simulink model "step_input_Q3_standard"  (R2023a)
settings: Solver=VariableStepAuto  StartTime=0.0  StopTime=50  RelTol=1e-3
libraries: simulink_extras x2
settings Model: Creator=anshu  LastModifiedBy=anshu

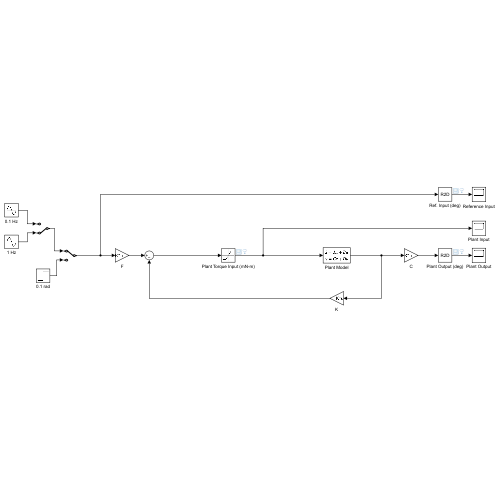
[thumbnail: Simulink's stored preview of the top-level diagram]
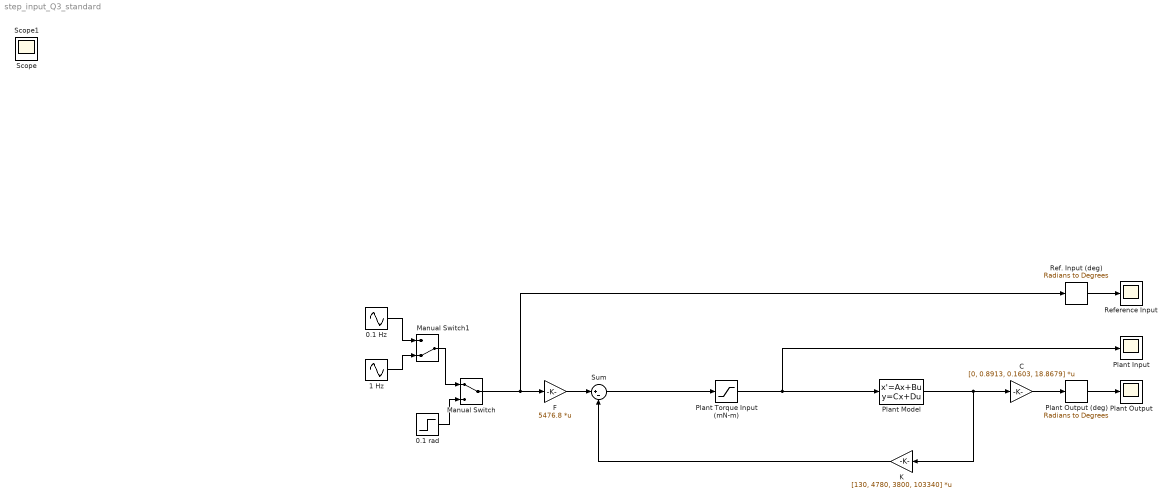
== system step_input_Q3_standard ==
  0.1 Hz : Sin  Amplitude=2.5  Frequency=0.628  SampleTime=0
  0.1 rad : Step  After=0.1  SampleTime=0
  1 Hz : Sin  Amplitude=0.3  Frequency=6.28  SampleTime=0
  C : Gain  Gain=[0, 0.8913, 0.1603, 18.8679]  Multiplication=Matrix(K*u)
  F : Gain  Gain=5476.8  Multiplication=Matrix(K*u)
  K : Gain  Gain=[130, 4780, 3800, 103340]  Multiplication=Matrix(K*u)
  Manual Switch : ManualSwitch
  Manual Switch1 : ManualSwitch  CurrentSetting=0
  Plant Input : Scope
  Plant Model : StateSpace  A=[-5.2954, -70.1022, -343.1258, 0; 1, 0, 0, 0; 0, 1, 0, 0; 0, 0, 1, 0]  B=[1; 0; 0; 0]  C=eye(4)  D=zeros(4,1)  InitialCondition=0  ParameterTunability=Unconstrained
  Plant Output : Scope
  Plant Output (deg) : simulink_extras/Transformations/Radians to Degrees
  Plant Torque Input (mN-m) : Saturate  UpperLimit=67  LowerLimit=-67
  Ref. Input (deg) : simulink_extras/Transformations/Radians to Degrees
  Reference Input : Scope
  Sum : Sum  Inputs=|+-
  Scope : Scope
  Scope1 : Scope
  wires:
  F/1 -> Sum/1
  Sum/1 -> Plant Torque Input (mN-m)/1
  Plant Model/1 -> C/1, K/1
  K/1 -> Sum/2
  Plant Torque Input (mN-m)/1 -> Plant Input/1, Plant Model/1
  C/1 -> Plant Output (deg)/1
  Plant Output (deg)/1 -> Plant Output/1
  Ref. Input (deg)/1 -> Reference Input/1
  Manual Switch/1 -> Ref. Input (deg)/1, F/1
  0.1 Hz/1 -> Manual Switch1/1
  1 Hz/1 -> Manual Switch1/2
  Manual Switch1/1 -> Manual Switch/1
  0.1 rad/1 -> Manual Switch/2
